simulink model "HVDCMTGW"  (R2025b)
settings: Solver=VariableStepAuto  StartTime=0.0  StopTime=Tsim  FixedStep=5e-5  RelTol=1e-3
PreLoadFcn:
  | SimulationTime = 3.5;
  | HVDCParameters;
  | Tsim = 3.5;
undefined symbols (not defined in the file): base, Base, Connection1, Connection2, Connection3, DiscIntNeverNeededParam, ee_sli_rtmsupport, frt, gcbh, grid, HVDC, lvrt, onshoreGfm, pll, pmsm, PVController, time, Ts, windController, windTransformer, windTurbine
libraries: fl_lib x51, ee_lib x46, nesl_utility x41, simulink x18, eeGeneralControl x12, eeTransforms x6
(part 1 of 4)
settings Model: SimulationMode=accelerator  Creator=Rajarshi  LastModifiedBy=rajarshd
settings SolverCC: AutoInsertRateTranBlk=on
settings DataIOCC: SaveOutput=off  DSMLogging=off  ReturnWorkspaceOutputsName=Data

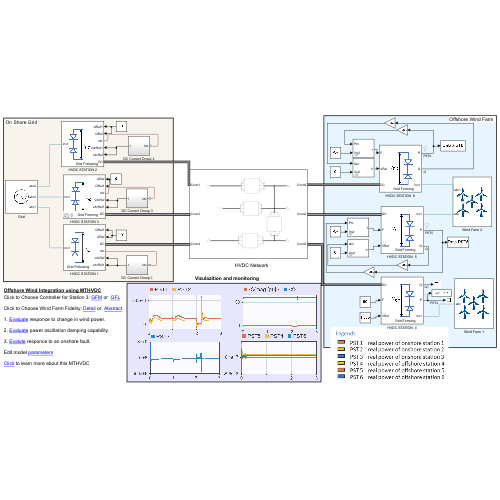
[thumbnail: Simulink's stored preview of the top-level diagram]
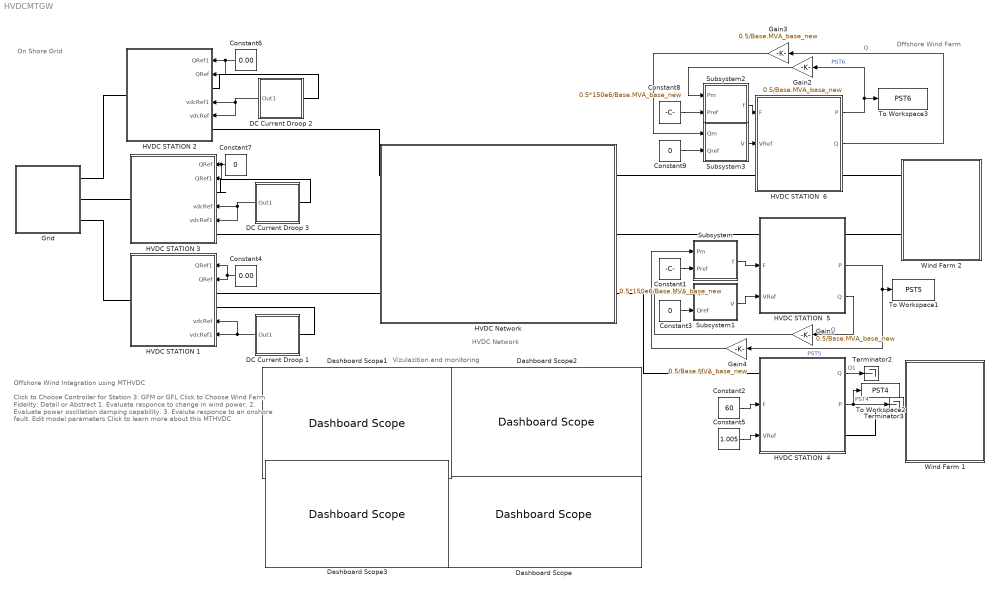
== system HVDCMTGW ==
  note: HVDC Network
  note: Click to Choose Controller for Station 3: GFM or GFL
      |
      | Click to Choose Wind Farm Fidelity: Detail or Abstract
      |
      | 1. Evaluate responce to change in wind power.
      |
      | 2. Evaluate power oscillation damping capability.
      |
      | 3. Evalute responce to an onshore fault.
      |
      | Edit model parameters
      |
      | Click to learn more about this MTHVDC
  note: Offshore Wind Integration using MTHVDC
  note: Offshore Wind Farm
  note: On Shore Grid
  note: Vizulazition and monitoring
  Constant1 : Constant  Value=0.5*150e6/Base.MVA_base_new
  Constant2 : Constant  Value=60
  Constant3 : Constant  Value=0
  Constant4 : Constant  Value=0.00
  Constant5 : Constant  Value=1.005
  Constant6 : Constant  Value=0.00
  Constant7 : Constant  Value=0
  Constant8 : Constant  Value=0.5*150e6/Base.MVA_base_new
  Constant9 : Constant  Value=0
  DC Current Droop 1 : Subsystem
  DC Current Droop 2 : Subsystem
  DC Current Droop 3 : Subsystem
  Dashboard Scope{,1..3} (4 alike) : DashboardScope  FontColor=[0.0, 0.0, 0.0]
  Gain{1..4} (4 alike) : Gain  Gain=0.5/Base.MVA_base_new
  Grid : Subsystem
  HVDC Network : Subsystem
  HVDC STATION  4 : Subsystem
      settings: PortSchema="{\"entries\":[{\"content\":{\"sides\":[{\"content\":{\"connectorIds\":[\"LConn1\",\"In1\",\"In2\"]},\"type\":\"ConnectorPlacement.EquallySpacedRectSide\",\"uuid\":\"6966c343-33fe-49bf-a40f-735765742aa3\"},{\"content\":{\"connectorIds\":[\"Out1\",\"Out2\",\"RConn1\"],\"side\":\"RIGHT\"},\"type\":\"ConnectorPlacement.EquallySpacedRectSide\",\"uuid\":\"561f8608-e59c-4a25-b590-fef3ac618496\"},{\"content\":{\"side\":\"TOP\"},\"type\":\"ConnectorPlacement.EquallySpacedRectSide\",\"uuid\":\"8731cc78-5557-4266-b8ae-4cd94a3cb230\"}]},\"type\":\"ConnectorPlacement.EquallySpacedConnector\",\"uuid\":\"a72f596e-11e5-4094-bfc9-f49a91172650\"}],\"packageUris\":[\"http://schema.mathworks.com/mf0/Connector/R2020b\"],\"version\":\"1.0\"}"
      mask Display:
      | text(40,10, 'Grid Forming');
      | image('HVDCstation.png', [0,0,0,0,80,80]);
  HVDC STATION  5 : Subsystem
      settings: PortSchema="{\"entries\":[{\"content\":{\"sides\":[{\"content\":{\"connectorIds\":[\"LConn1\",\"In1\",\"In2\"]},\"type\":\"ConnectorPlacement.EquallySpacedRectSide\",\"uuid\":\"42fca73d-9b1c-4b14-af1d-17a95f3928f9\"},{\"content\":{\"connectorIds\":[\"RConn1\",\"Out1\",\"Out2\"],\"side\":\"RIGHT\"},\"type\":\"ConnectorPlacement.EquallySpacedRectSide\",\"uuid\":\"9128ed72-a507-450a-8a5b-bb565d329306\"},{\"content\":{\"side\":\"TOP\"},\"type\":\"ConnectorPlacement.EquallySpacedRectSide\",\"uuid\":\"7e656d19-2b54-419b-9669-320b071747a0\"}]},\"type\":\"ConnectorPlacement.EquallySpacedConnector\",\"uuid\":\"734da2a5-0bfe-48f8-afaf-e709645445a8\"}],\"packageUris\":[\"http://schema.mathworks.com/mf0/Connector/R2020b\"],\"version\":\"1.0\"}"
      mask Display:
      | text(40,10, 'Grid Forming');
      | image('HVDCstation.png', [0,0,0,0,80,80]);
  HVDC STATION  6 : Subsystem
      mask Display:
      | text(40,10, 'Grid Forming');
      | image('HVDCstation.png', [0,0,0,0,80,80]);
  HVDC STATION 1 : Subsystem
      settings: PortSchema="{\"entries\":[{\"content\":{\"sides\":[{\"content\":{\"connectorIds\":[\"In1\",\"In2\",\"LConn1\",\"LConn2\",\"In3\",\"In4\"]},\"type\":\"ConnectorPlacement.EquallySpacedRectSide\",\"uuid\":\"825870e3-6597-48fb-b44e-9cac78187e1c\"},{\"content\":{\"connectorIds\":[\"RConn1\"],\"side\":\"RIGHT\"},\"type\":\"ConnectorPlacement.EquallySpacedRectSide\",\"uuid\":\"0ccf2e17-8e04-4158-8531-c061fa3c835c\"},{\"content\":{\"side\":\"TOP\"},\"type\":\"ConnectorPlacement.EquallySpacedRectSide\",\"uuid\":\"f5f3d6c6-bb99-4c25-841e-4b6e2b2ba3c2\"}]},\"type\":\"ConnectorPlacement.EquallySpacedConnector\",\"uuid\":\"7882ba9b-b66e-421c-89fd-6c0e858bc84c\"}],\"packageUris\":[\"http://schema.mathworks.com/mf0/Connector/R2020b\"],\"version\":\"1.0\"}"
      mask Display:
      | text(10,10, 'Grid Following');
      | image('HVDCstation1.png', [0,2,12,2,80,80]);
  HVDC STATION 2 : Subsystem
      settings: PortSchema="{\"entries\":[{\"content\":{\"sides\":[{\"content\":{\"connectorIds\":[\"In1\",\"In2\",\"LConn1\",\"In3\",\"In4\",\"LConn2\"]},\"type\":\"ConnectorPlacement.EquallySpacedRectSide\",\"uuid\":\"ae8d0010-9935-44cd-9427-2860d952f744\"},{\"content\":{\"connectorIds\":[\"RConn1\"],\"side\":\"RIGHT\"},\"type\":\"ConnectorPlacement.EquallySpacedRectSide\",\"uuid\":\"5b1bea21-e058-4721-9c71-335e968af1dc\"},{\"content\":{\"side\":\"TOP\"},\"type\":\"ConnectorPlacement.EquallySpacedRectSide\",\"uuid\":\"e2b4b649-cbe9-452b-9e7c-c313a834e66c\"}]},\"type\":\"ConnectorPlacement.EquallySpacedConnector\",\"uuid\":\"ef58559f-fad3-48cf-8f32-7426dfcc4f07\"}],\"packageUris\":[\"http://schema.mathworks.com/mf0/Connector/R2020b\"],\"version\":\"1.0\"}"
      mask Display:
      | text(40,10, 'Grid Following');
      | image('HVDCstation1.png', [0,2,12,2,80,80]);
  HVDC STATION 3 : Subsystem  Variant=on  mask{Choice=GFM}
      mask prompts: Choice "Controller"
      settings: PortSchema="{\"entries\":[{\"content\":{\"sides\":[{\"content\":{\"connectorIds\":[\"In1\",\"In2\",\"LConn1\",\"In3\",\"In4\",\"LConn2\"]},\"type\":\"ConnectorPlacement.EquallySpacedRectSide\",\"uuid\":\"ae8d0010-9935-44cd-9427-2860d952f744\"},{\"content\":{\"connectorIds\":[\"RConn1\"],\"side\":\"RIGHT\"},\"type\":\"ConnectorPlacement.EquallySpacedRectSide\",\"uuid\":\"5b1bea21-e058-4721-9c71-335e968af1dc\"},{\"content\":{\"side\":\"TOP\"},\"type\":\"ConnectorPlacement.EquallySpacedRectSide\",\"uuid\":\"e2b4b649-cbe9-452b-9e7c-c313a834e66c\"}]},\"type\":\"ConnectorPlacement.EquallySpacedConnector\",\"uuid\":\"ef58559f-fad3-48cf-8f32-7426dfcc4f07\"}],\"packageUris\":[\"http://schema.mathworks.com/mf0/Connector/R2020b\"],\"version\":\"1.0\"}"
  Subsystem : Subsystem  mask{kp=0.02, t=5e-3, f=60}
      mask prompts: kp "Frequency Droop (PU)"; t "Filter Time Constant (sec)"; f "Reference Frequency (Hz)"
  Subsystem1 : Subsystem  mask{kq=0.02, t=5e-3, V=1.005}
      mask prompts: kq "Voltage Droop (PU)"; t "Filter Time Constant (sec)"; V "Voltage Reference (PU)"
  Subsystem2 : Subsystem  mask{kp=0.01, t=5e-3, f=60}
      mask prompts: kp "Frequency Droop (PU)"; t "Filter Time Constant (sec)"; f "Reference Frequency (Hz)"
  Subsystem3 : Subsystem  mask{kq=0.01, t=5e-3, V=1.005}
      mask prompts: kq "Voltage Droop (PU)"; t "Filter Time Constant (sec)"; V "Voltage Reference (PU)"
  Terminator2 : Terminator
  Terminator3 : Terminator
  To Workspace1 : ToWorkspace  VariableName=PST5  SaveFormat=Timeseries  SampleTime=-1
  To Workspace2 : ToWorkspace  VariableName=PST4  SaveFormat=Timeseries  SampleTime=-1
  To Workspace3 : ToWorkspace  VariableName=PST6  SaveFormat=Timeseries  SampleTime=-1
  Wind Farm 1 : Subsystem
      mask Display: image('Windfirm3.png', [0,0,0,0,80,80]);
  Wind Farm 2 : Subsystem
      mask Display: image('Windfirm3.png', [0,0,0,0,80,80]);
  wires:
  Constant5/1 -> HVDC STATION  4/2(VRef)
  HVDC STATION  4/1(Q) -> Terminator2/1  "Q1"
  Constant2/1 -> HVDC STATION  4/1(F)
  HVDC STATION  4/2(P) -> Terminator3/1, To Workspace2/1  "PST4"
  Constant7/1 -> HVDC STATION 3/1(QRef), HVDC STATION 3/2(QRef1)
  DC Current Droop 1/1(Out1) -> HVDC STATION 1/3(vdcRef), HVDC STATION 1/4(vdcRef1)
  Constant4/1 -> HVDC STATION 1/1(QRef1), HVDC STATION 1/2(QRef)
  Constant6/1 -> HVDC STATION 2/2(QRef), HVDC STATION 2/1(QRef1)
  DC Current Droop 2/1(Out1) -> HVDC STATION 2/4(vdcRef), HVDC STATION 2/3(vdcRef1)
  Constant1/1 -> Subsystem/2(Pref)
  Constant3/1 -> Subsystem1/2(Qref)
  Constant8/1 -> Subsystem2/2(Pref)
  HVDC STATION  6/1(P) -> To Workspace3/1, Gain2/1  "PST6"
  Subsystem3/1(V) -> HVDC STATION  6/2(VRef)
  Subsystem2/1(f) -> HVDC STATION  6/1(F)
  HVDC STATION  6/2(Q) -> Gain3/1  "Q"
  Constant9/1 -> Subsystem3/2(Qref)
  Gain3/1 -> Subsystem3/1(Qm)
  Gain2/1 -> Subsystem2/1(Pm)
  Subsystem/1(f) -> HVDC STATION  5/1(F)
  Subsystem1/1(V) -> HVDC STATION  5/2(VRef)
  HVDC STATION  5/2(Q) -> Gain1/1  "Q"
  HVDC STATION  5/1(P) -> To Workspace1/1, Gain4/1  "PST5"
  Gain1/1 -> Subsystem1/1(Qm)
  Gain4/1 -> Subsystem/1(Pm)
  DC Current Droop 3/1(Out1) -> HVDC STATION 3/3(vdcRef), HVDC STATION 3/4(vdcRef1)
  connections:
  Wind Farm 2/RConn2 -- HVDC STATION  5/RConn1
  HVDC STATION 3/LConn2 -- HVDC Network/RConn2
  HVDC Network/LConn3 -- HVDC STATION  4/LConn1
  HVDC STATION 1/LConn1 -- HVDC Network/RConn3
  Grid/RConn3 -- HVDC STATION 1/RConn1
  DC Current Droop 1/LConn1 -- HVDC STATION 1/LConn2
  DC Current Droop 2/LConn1 -- HVDC STATION 2/LConn1
  HVDC STATION 2/LConn2 -- HVDC Network/RConn1
  Grid/RConn1 -- HVDC STATION 2/RConn1
  HVDC STATION  6/RConn1 -- Wind Farm 2/RConn1
  HVDC STATION  6/LConn1 -- HVDC Network/LConn1
  Wind Farm 1/RConn1 -- HVDC STATION  4/RConn1
  HVDC STATION 3/LConn1 -- DC Current Droop 3/LConn1
  HVDC STATION  5/LConn1 -- HVDC Network/LConn2
  HVDC STATION 3/RConn1 -- Grid/RConn2

== system HVDCMTGW/DC Current Droop 1 ==
  Constant : Constant  Value=HVDC.Vdc
  Gain : Gain  Gain=0.04
  Gain1 : Gain  Gain=2
  PS-Simulink Converter : nesl_utility/PS-Simulink Converter  PhysicalDomain=network_engine_domain  SubClassName=ps_output  LeftPortType=input  RightPortType=output  PseudoPeriodic=off  Frequencies=[]  VectorFormat=inherit  Unit=inherit  AffineConversion=off
  Sum : Sum  Inputs=|++
  Terminator1 : Terminator
  Unit Delay9 : UnitDelay  SampleTime=-1  HasFrameUpgradeWarning=on
  Idc : PMIOPort  Side=Left
  Out1 : Outport
  wires:
  Gain/1 -> Sum/1
  Unit Delay9/1 -> Gain/1
  Constant/1 -> Sum/2
  PS-Simulink Converter/1 -> Unit Delay9/1
  Sum/1 -> Gain1/1, Out1/1
  Gain1/1 -> Terminator1/1  "VdcRef"
  connections:
  Idc/RConn1 -- PS-Simulink Converter/LConn1

== system HVDCMTGW/DC Current Droop 2 ==
  Constant : Constant  Value=HVDC.Vdc
  Gain : Gain  Gain=0.01
  Gain1 : Gain  Gain=2
  PS-Simulink Converter : nesl_utility/PS-Simulink Converter  PhysicalDomain=network_engine_domain  SubClassName=ps_output  LeftPortType=input  RightPortType=output  PseudoPeriodic=off  Frequencies=[]  VectorFormat=inherit  Unit=inherit  AffineConversion=off
  Sum : Sum  Inputs=|++
  Terminator1 : Terminator
  Unit Delay9 : UnitDelay  SampleTime=-1  HasFrameUpgradeWarning=on
  Idc : PMIOPort  Side=Left
  Out1 : Outport
  wires:
  Gain/1 -> Sum/1
  Unit Delay9/1 -> Gain/1
  Constant/1 -> Sum/2
  PS-Simulink Converter/1 -> Unit Delay9/1
  Sum/1 -> Gain1/1, Out1/1
  Gain1/1 -> Terminator1/1  "VdcRef"
  connections:
  Idc/RConn1 -- PS-Simulink Converter/LConn1

== system HVDCMTGW/DC Current Droop 3 ==
  Constant : Constant  Value=HVDC.Vdc
  Gain : Gain  Gain=0.01
  Gain1 : Gain  Gain=2
  PS-Simulink Converter : nesl_utility/PS-Simulink Converter  PhysicalDomain=network_engine_domain  SubClassName=ps_output  LeftPortType=input  RightPortType=output  PseudoPeriodic=off  Frequencies=[]  VectorFormat=inherit  Unit=inherit  AffineConversion=off
  Sum : Sum  Inputs=|++
  Terminator1 : Terminator
  Unit Delay9 : UnitDelay  SampleTime=-1  HasFrameUpgradeWarning=on
  Idc : PMIOPort  Side=Left
  Out1 : Outport
  wires:
  Gain/1 -> Sum/1
  Unit Delay9/1 -> Gain/1
  Constant/1 -> Sum/2
  PS-Simulink Converter/1 -> Unit Delay9/1
  Sum/1 -> Gain1/1, Out1/1
  Gain1/1 -> Terminator1/1  "VdcRef"
  connections:
  Idc/RConn1 -- PS-Simulink Converter/LConn1

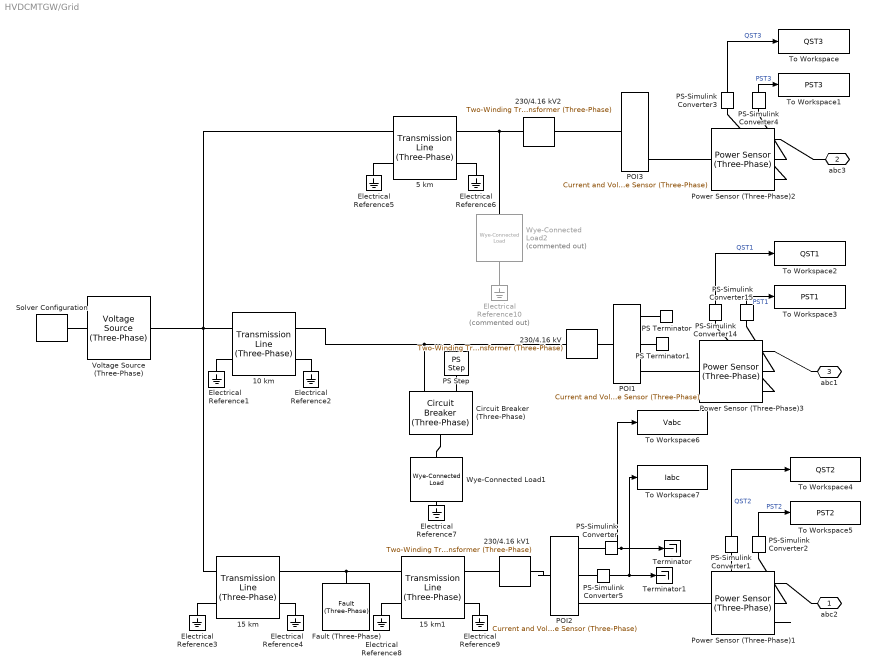
== system HVDCMTGW/Grid ==
  10 km : ee_lib/Passive/Lines/Transmission Line (Three-Phase)  length=10 km  freq=60 Hz  R=0.02 Ohm/km  L=0.5 mH/km  M=0.1 mH/km  Cl=0.3 uF/km  Cg=0.1 uF/km  Rm=0 Ohm/km  ModelTwoSections=ee.enum.enable.no  N=1  InterfacePosition=0.5 km  N1sec=1  N2sec=1  Access_ground=ee.enum.enable.no  R_parasitic=1e-6 Ohm  G_parasitic=1e-6 1/Ohm
      settings: InternalSimscapePortConfiguration="{\"Bottom\":[],\"Left\":[{\"id\":\"N1\",\"label\":\"~1\",\"type\":\"foundation.electrical.three_phase\"},{\"id\":\"g1\",\"label\":\"g1\",\"type\":\"foundation.electrical.electrical\"}],\"Right\":[{\"id\":\"N2\",\"label\":\"~2\",\"type\":\"foundation.electrical.three_phase\"},{\"id\":\"g2\",\"label\":\"g2\",\"type\":\"foundation.electrical.electrical\"}],\"Top\":[]}"
  15 km : ee_lib/Passive/Lines/Transmission Line (Three-Phase)  length=15 km  freq=60 Hz  R=0.02 Ohm/km  L=0.5 mH/km  M=0.1 mH/km  Cl=0.3 uF/km  Cg=0.1 uF/km  Rm=0 Ohm/km  ModelTwoSections=ee.enum.enable.no  N=1  InterfacePosition=0.5 km  N1sec=1  N2sec=1  Access_ground=ee.enum.enable.no  R_parasitic=1e-6 Ohm  G_parasitic=1e-6 1/Ohm
      settings: InternalSimscapePortConfiguration="{\"Bottom\":[],\"Left\":[{\"id\":\"N1\",\"label\":\"~1\",\"type\":\"foundation.electrical.three_phase\"},{\"id\":\"g1\",\"label\":\"g1\",\"type\":\"foundation.electrical.electrical\"}],\"Right\":[{\"id\":\"N2\",\"label\":\"~2\",\"type\":\"foundation.electrical.three_phase\"},{\"id\":\"g2\",\"label\":\"g2\",\"type\":\"foundation.electrical.electrical\"}],\"Top\":[]}"
  15 km1 : ee_lib/Passive/Lines/Transmission Line (Three-Phase)  length=15 km  freq=60 Hz  R=0.02 Ohm/km  L=0.5 mH/km  M=0.1 mH/km  Cl=0.3 uF/km  Cg=0.1 uF/km  Rm=0 Ohm/km  ModelTwoSections=ee.enum.enable.no  N=1  InterfacePosition=0.5 km  N1sec=1  N2sec=1  Access_ground=ee.enum.enable.no  R_parasitic=1e-6 Ohm  G_parasitic=1e-6 1/Ohm
      settings: InternalSimscapePortConfiguration="{\"Bottom\":[],\"Left\":[{\"id\":\"N1\",\"label\":\"~1\",\"type\":\"foundation.electrical.three_phase\"},{\"id\":\"g1\",\"label\":\"g1\",\"type\":\"foundation.electrical.electrical\"}],\"Right\":[{\"id\":\"N2\",\"label\":\"~2\",\"type\":\"foundation.electrical.three_phase\"},{\"id\":\"g2\",\"label\":\"g2\",\"type\":\"foundation.electrical.electrical\"}],\"Top\":[]}"
  230/4.16 kV : ee_lib/Passive/Transformers/Two-Winding Transformer (Three-Phase)  SRated=windTransformer.va A*V  FRated=grid.frequency Hz  Winding1Connection=ee.enum.windingconnection.Yg  VRated1=windTransformer.hv*1.25 V  Winding2Connection=ee.enum.windingconnection.Yg  VRated2=base.kV V  CoreType=ee.enum.coretype.threelimb  pu_Rw1=windTransformer.windingResistance/20  pu_Rw2=windTransformer.windingResistance/20  leakage_reactance_option=ee.enum.transformer_leakage.include  pu_Xl1=windTransformer.windingLekageReactance/20  pu_Xl2=windTransformer.windingLekageReactance/20  magnetizing_resistance_option=ee.enum.transformer_magnetizingResistance.exclude  pu_Rm=500  magnetizing_reactance_option=ee.enum.transformer_magnetizingReactance.exclude  saturation_option=ee.enum.transformer_saturation.exclude  pu_Xm=500  current_data=[0, .002, 1, 2]  magnetic_flux_data=[0, 1.2, 1.5, 1.51]  pu_X0=windTransformer.zeroSequenceReactance  i1_specify=off  i1_priority=None  i1=[0, 0, 0] A  i1_nominal_specify=off  i1_nominal_value=1  i1_nominal_unit=A  i2_specify=off  i2_priority=None  i2=[0, 0, 0] A  i2_nominal_specify=off  i2_nominal_value=1  i2_nominal_unit=A  phi_specify=off  phi_priority=None  phi=[0, 0, 0]  phi_nominal_specify=off  phi_nominal_value=1  phi_nominal_unit=1  power_dissipated_specify=off  power_dissipated_priority=None  power_dissipated=0 W  power_dissipated_nominal_specify=off  power_dissipated_nominal_value=1  power_dissipated_nominal_unit=W
      settings: InternalSimscapePortConfiguration="{\"Bottom\":[],\"Left\":[{\"id\":\"N1\",\"label\":\"~1\",\"type\":\"foundation.electrical.three_phase\"}],\"Right\":[{\"id\":\"N2\",\"label\":\"~2\",\"type\":\"foundation.electrical.three_phase\"}],\"Top\":[]}"
  230/4.16 kV1 : ee_lib/Passive/Transformers/Two-Winding Transformer (Three-Phase)  SRated=windTransformer.va A*V  FRated=grid.frequency Hz  Winding1Connection=ee.enum.windingconnection.Yg  VRated1=windTransformer.hv*1.25 V  Winding2Connection=ee.enum.windingconnection.Yg  VRated2=base.kV V  CoreType=ee.enum.coretype.threelimb  pu_Rw1=windTransformer.windingResistance/20  pu_Rw2=windTransformer.windingResistance/20  leakage_reactance_option=ee.enum.transformer_leakage.include  pu_Xl1=windTransformer.windingLekageReactance/20  pu_Xl2=windTransformer.windingLekageReactance/20  magnetizing_resistance_option=ee.enum.transformer_magnetizingResistance.exclude  pu_Rm=500  magnetizing_reactance_option=ee.enum.transformer_magnetizingReactance.exclude  saturation_option=ee.enum.transformer_saturation.exclude  pu_Xm=500  current_data=[0, .002, 1, 2]  magnetic_flux_data=[0, 1.2, 1.5, 1.51]  pu_X0=windTransformer.zeroSequenceReactance  i1_specify=off  i1_priority=None  i1=[0, 0, 0] A  i1_nominal_specify=off  i1_nominal_value=1  i1_nominal_unit=A  i2_specify=off  i2_priority=None  i2=[0, 0, 0] A  i2_nominal_specify=off  i2_nominal_value=1  i2_nominal_unit=A  phi_specify=off  phi_priority=None  phi=[0, 0, 0]  phi_nominal_specify=off  phi_nominal_value=1  phi_nominal_unit=1  power_dissipated_specify=off  power_dissipated_priority=None  power_dissipated=0 W  power_dissipated_nominal_specify=off  power_dissipated_nominal_value=1  power_dissipated_nominal_unit=W
      settings: InternalSimscapePortConfiguration="{\"Bottom\":[],\"Left\":[{\"id\":\"N1\",\"label\":\"~1\",\"type\":\"foundation.electrical.three_phase\"}],\"Right\":[{\"id\":\"N2\",\"label\":\"~2\",\"type\":\"foundation.electrical.three_phase\"}],\"Top\":[]}"
  230/4.16 kV2 : ee_lib/Passive/Transformers/Two-Winding Transformer (Three-Phase)  SRated=windTransformer.va A*V  FRated=grid.frequency Hz  Winding1Connection=ee.enum.windingconnection.Yg  VRated1=windTransformer.hv*1.25 V  Winding2Connection=ee.enum.windingconnection.Yg  VRated2=base.kV V  CoreType=ee.enum.coretype.threelimb  pu_Rw1=windTransformer.windingResistance/20  pu_Rw2=windTransformer.windingResistance/20  leakage_reactance_option=ee.enum.transformer_leakage.include  pu_Xl1=windTransformer.windingLekageReactance/20  pu_Xl2=windTransformer.windingLekageReactance/20  magnetizing_resistance_option=ee.enum.transformer_magnetizingResistance.exclude  pu_Rm=500  magnetizing_reactance_option=ee.enum.transformer_magnetizingReactance.exclude  saturation_option=ee.enum.transformer_saturation.exclude  pu_Xm=500  current_data=[0, .002, 1, 2]  magnetic_flux_data=[0, 1.2, 1.5, 1.51]  pu_X0=windTransformer.zeroSequenceReactance  i1_specify=off  i1_priority=None  i1=[0, 0, 0] A  i1_nominal_specify=off  i1_nominal_value=1  i1_nominal_unit=A  i2_specify=off  i2_priority=None  i2=[0, 0, 0] A  i2_nominal_specify=off  i2_nominal_value=1  i2_nominal_unit=A  phi_specify=off  phi_priority=None  phi=[0, 0, 0]  phi_nominal_specify=off  phi_nominal_value=1  phi_nominal_unit=1  power_dissipated_specify=off  power_dissipated_priority=None  power_dissipated=0 W  power_dissipated_nominal_specify=off  power_dissipated_nominal_value=1  power_dissipated_nominal_unit=W
      settings: InternalSimscapePortConfiguration="{\"Bottom\":[],\"Left\":[{\"id\":\"N1\",\"label\":\"~1\",\"type\":\"foundation.electrical.three_phase\"}],\"Right\":[{\"id\":\"N2\",\"label\":\"~2\",\"type\":\"foundation.electrical.three_phase\"}],\"Top\":[]}"
  5 km : ee_lib/Passive/Lines/Transmission Line (Three-Phase)  length=5 km  freq=60 Hz  R=0.02 Ohm/km  L=0.5 mH/km  M=0.1 mH/km  Cl=0.3 uF/km  Cg=0.1 uF/km  Rm=0 Ohm/km  ModelTwoSections=ee.enum.enable.no  N=1  InterfacePosition=0.5 km  N1sec=1  N2sec=1  Access_ground=ee.enum.enable.no  R_parasitic=1e-6 Ohm  G_parasitic=1e-6 1/Ohm
      settings: InternalSimscapePortConfiguration="{\"Bottom\":[],\"Left\":[{\"id\":\"N1\",\"label\":\"~1\",\"type\":\"foundation.electrical.three_phase\"},{\"id\":\"g1\",\"label\":\"g1\",\"type\":\"foundation.electrical.electrical\"}],\"Right\":[{\"id\":\"N2\",\"label\":\"~2\",\"type\":\"foundation.electrical.three_phase\"},{\"id\":\"g2\",\"label\":\"g2\",\"type\":\"foundation.electrical.electrical\"}],\"Top\":[]}"
  Circuit Breaker (Three-Phase) : ee_lib/Switches & Breakers/Circuit Breaker (Three-Phase)  R_closed=1e-7 Ohm  G_open=1e-6 1/Ohm  threshold=0.5 V  breaker_behavior=ee.enum.switches.breakerBehavior.zeroCrossingDisable
      settings: InternalSimscapePortConfiguration="{\"Bottom\":[],\"Left\":[{\"id\":\"vT\",\"label\":\"vT\",\"type\":\"input\"},{\"id\":\"N1\",\"label\":\"~1\",\"type\":\"foundation.electrical.three_phase\"}],\"Right\":[{\"id\":\"N2\",\"label\":\"~2\",\"type\":\"foundation.electrical.three_phase\"}],\"Top\":[]}"
  Electrical Reference{1..9} (9 alike) : fl_lib/Electrical/Electrical Elements/Electrical Reference
  Electrical Reference10 : fl_lib/Electrical/Electrical Elements/Electrical Reference  Commented=on
  Fault (Three-Phase) : ee_lib/Utilities/Fault (Three-Phase)  fault_type_option=11  R_pn_fault=1e-6 Ohm  R_ng_fault=1e-6 Ohm  exposemeasurement=ee.enum.exposemeasurement.hidden  enable_external_fault=ee.enum.external_fault.hidden  fault_threshold=0.5  fault_condition=1  fault_resettable=0  enable_temporal_fault=1  fault_start_time=time.fault s  fault_duration=0.2 s  G_parasitic=1e-6 1/Ohm
      settings: InternalSimscapePortConfiguration="{\"Bottom\":[],\"Left\":[{\"id\":\"N\",\"label\":\"~\",\"type\":\"foundation.electrical.three_phase\"}],\"Right\":[],\"Top\":[]}"
  POI1 : ee_lib/Sensors & Transducers/Current and Voltage Sensor (Three-Phase)  vMeasurementType=ee.enum.vmeasurement.lg  outputUnit=ee.enum.unit.pu  SRated=Base.MVA_base_new A*V  VRated=base.kV V  I_specify=off  I_priority=None  I=[0, 0, 0] A  I_nominal_specify=off  I_nominal_value=1  I_nominal_unit=A  V_specify=off  V_priority=None  V=[0, 0, 0] V  V_nominal_specify=off  V_nominal_value=1  V_nominal_unit=V
      settings: InternalSimscapePortConfiguration="{\"Bottom\":[],\"Left\":[{\"id\":\"N1\",\"label\":\"~1\",\"type\":\"foundation.electrical.three_phase\"}],\"Right\":[{\"id\":\"V_output\",\"label\":\"V\",\"type\":\"output\"},{\"id\":\"I_output\",\"label\":\"I\",\"type\":\"output\"},{\"id\":\"N2\",\"label\":\"~2\",\"type\":\"foundation.electrical.three_phase\"}],\"Top\":[]}"
  POI2 : ee_lib/Sensors & Transducers/Current and Voltage Sensor (Three-Phase)  vMeasurementType=ee.enum.vmeasurement.lg  outputUnit=ee.enum.unit.pu  SRated=Base.MVA_base_new A*V  VRated=base.kV V  I_specify=off  I_priority=None  I=[0, 0, 0] A  I_nominal_specify=off  I_nominal_value=1  I_nominal_unit=A  V_specify=off  V_priority=None  V=[0, 0, 0] V  V_nominal_specify=off  V_nominal_value=1  V_nominal_unit=V
      settings: InternalSimscapePortConfiguration="{\"Bottom\":[],\"Left\":[{\"id\":\"N1\",\"label\":\"~1\",\"type\":\"foundation.electrical.three_phase\"}],\"Right\":[{\"id\":\"V_output\",\"label\":\"V\",\"type\":\"output\"},{\"id\":\"I_output\",\"label\":\"I\",\"type\":\"output\"},{\"id\":\"N2\",\"label\":\"~2\",\"type\":\"foundation.electrical.three_phase\"}],\"Top\":[]}"
  POI3 : ee_lib/Sensors & Transducers/Current and Voltage Sensor (Three-Phase)  vMeasurementType=ee.enum.vmeasurement.lg  outputUnit=ee.enum.unit.pu  SRated=Base.MVA_base_new A*V  VRated=base.kV V  I_specify=off  I_priority=None  I=[0, 0, 0] A  I_nominal_specify=off  I_nominal_value=1  I_nominal_unit=A  V_specify=off  V_priority=None  V=[0, 0, 0] V  V_nominal_specify=off  V_nominal_value=1  V_nominal_unit=V
      settings: InternalSimscapePortConfiguration="{\"Bottom\":[],\"Left\":[{\"id\":\"N1\",\"label\":\"~1\",\"type\":\"foundation.electrical.three_phase\"}],\"Right\":[{\"id\":\"V_output\",\"label\":\"V\",\"type\":\"output\"},{\"id\":\"I_output\",\"label\":\"I\",\"type\":\"output\"},{\"id\":\"N2\",\"label\":\"~2\",\"type\":\"foundation.electrical.three_phase\"}],\"Top\":[]}"
  PS Step : fl_lib/Physical Signals/Sources/PS Step  step_time=time.load s  initial_value=0  final_value=1
  PS Terminator : fl_lib/Physical Signals/Sinks/PS Terminator
  PS Terminator1 : fl_lib/Physical Signals/Sinks/PS Terminator
  PS-Simulink Converter{,1..5,14..15} (8 alike) : nesl_utility/PS-Simulink Converter  PhysicalDomain=network_engine_domain  SubClassName=ps_output  LeftPortType=input  RightPortType=output  PseudoPeriodic=off  Frequencies=[]  VectorFormat=inherit  Unit=inherit  AffineConversion=off
  Power Sensor (Three-Phase)1 : ee_lib/Sensors & Transducers/Power Sensor (Three-Phase)  load_type=ee.enum.passive.type_balanced.balanced  f0=60 Hz
      settings: InternalSimscapePortConfiguration="{\"Bottom\":[],\"Left\":[{\"id\":\"N1\",\"label\":\"~1\",\"type\":\"foundation.electrical.three_phase\"}],\"Right\":[{\"id\":\"N2\",\"label\":\"~2\",\"type\":\"foundation.electrical.three_phase\"}],\"Top\":[{\"id\":\"Pm\",\"label\":\"P\",\"type\":\"output\"},{\"id\":\"Qm\",\"label\":\"Q\",\"type\":\"output\"}]}"
  Power Sensor (Three-Phase)2 : ee_lib/Sensors & Transducers/Power Sensor (Three-Phase)  load_type=ee.enum.passive.type_balanced.balanced  f0=60 Hz
      settings: InternalSimscapePortConfiguration="{\"Bottom\":[],\"Left\":[{\"id\":\"N1\",\"label\":\"~1\",\"type\":\"foundation.electrical.three_phase\"}],\"Right\":[{\"id\":\"N2\",\"label\":\"~2\",\"type\":\"foundation.electrical.three_phase\"}],\"Top\":[{\"id\":\"Pm\",\"label\":\"P\",\"type\":\"output\"},{\"id\":\"Qm\",\"label\":\"Q\",\"type\":\"output\"}]}"
  Power Sensor (Three-Phase)3 : ee_lib/Sensors & Transducers/Power Sensor (Three-Phase)  load_type=ee.enum.passive.type_balanced.balanced  f0=60 Hz
      settings: InternalSimscapePortConfiguration="{\"Bottom\":[],\"Left\":[{\"id\":\"N1\",\"label\":\"~1\",\"type\":\"foundation.electrical.three_phase\"}],\"Right\":[{\"id\":\"N2\",\"label\":\"~2\",\"type\":\"foundation.electrical.three_phase\"}],\"Top\":[{\"id\":\"Pm\",\"label\":\"P\",\"type\":\"output\"},{\"id\":\"Qm\",\"label\":\"Q\",\"type\":\"output\"}]}"
  Solver Configuration : nesl_utility/Solver Configuration  PhysicalDomain=network_engine_domain  SubClassName=solver  LeftPortType=input  RightPortType=generic  Tones=[]  Harmonics=[]  SimulateNoise=off  Profile=off  UseLocalSampling=off  EnableSwitchedLinearOptims=on  FrequencyDomain=off  UseCCode=off  RelTol=0.001  AbsTol=0.001  MinStep=1e-09  ToWorkspace=off  RevertToSquareIcSolve=off  NumHomotopyIterations=100  PhasorMode=off  PhasorModeNumHarmonics=1  ConsistencySolver=NEWTON_XTOL_AFTER_FTOL  IndexReductionMethod=None  DoDC=off  ResidualTolerance=1e-09  ConsistencyTolSource=LOCAL  ConsistencyAbsTol=1e-3  ConsistencyRelTol=1e-3  ConsistencyTolFactor=1e-3  UseLocalSolver=on  LocalSolverChoice=NE_BACKWARD_EULER_ADVANCER  ResolveIndetEquations=off  FunctionEvalNumThread=1  LocalSolverSampleTime=5e-5  DoFixedCost=on  MaxNonlinIter=1  MaxModeIter=2  ComputeImpulses=off  ImpulseIterations=2  LinearAlgebra=Sparse  LinearAlgebraNumThread=0  EquationFormulation=NE_TIME_EF  DelaysMemoryBudget=1024  AutomaticFiltering=off  FilteringTimeConstant=0.001  PartitionStorageMethod=AS_NEEDED  PartitionMemoryBudget=1024  PartitionMethod=ROBUST  MultibodyUseLocalSolver=off  MultibodyLocalSolverChoice=ODE1  MultibodyLocalSolverSampleTime=0.001
  Terminator : Terminator
  Terminator1 : Terminator
  To Workspace : ToWorkspace  VariableName=QST3  SaveFormat=Timeseries  SampleTime=-1
  To Workspace1 : ToWorkspace  VariableName=PST3  SaveFormat=Timeseries  SampleTime=-1
  To Workspace2 : ToWorkspace  VariableName=QST1  SaveFormat=Timeseries  SampleTime=-1
  To Workspace3 : ToWorkspace  VariableName=PST1  SaveFormat=Timeseries  SampleTime=-1
  To Workspace4 : ToWorkspace  VariableName=QST2  SaveFormat=Timeseries  SampleTime=-1
  To Workspace5 : ToWorkspace  VariableName=PST2  SaveFormat=Timeseries  SampleTime=-1
  To Workspace6 : ToWorkspace  VariableName=Vabc  SaveFormat=Timeseries  SampleTime=-1
  To Workspace7 : ToWorkspace  VariableName=Iabc  SaveFormat=Timeseries  SampleTime=-1
  Voltage Source (Three-Phase) : ee_lib/Sources/Voltage Source (Three-Phase)  vline_rms=Grid.voltage V  shift=0 deg  freq=Grid.frequency Hz  impedance_option=4  SShortCircuit=1e6 A*V  XR=15  R=grid.rs*1.2 Ohm  L=grid.ls*1.2 H  harmonic_option=0  harmonic_orders=[5, 7, 11, 13]  harmonic_ratios=[.1, .1, .1, .1]  G_parasitic=1e-6 1/Ohm  I_specify=off  I_priority=None  I=[0, 0, 0] A  I_nominal_specify=off  I_nominal_value=1  I_nominal_unit=A
  Wye-Connected Load1 : ee_lib/Passive/RLC Assemblies/Wye-Connected Load  port_option=ee.enum.threePhasePort.composite  parameterization=ee.enum.rlc.parameterization.ratedpower  component_structure=ee.enum.rlc.structure.R  component_structure_PQ=ee.enum.rlc.structure.R  R=1 Ohm  L=1e-3 H  C=1e-6 F  VRated=230e3 V  FRated=60 Hz  P=300 MW  Qpos=100 A*V  Qneg=-1e2 A*V  R_parasitic=0 Ohm  G_parasitic=0 1/Ohm  R_parasitic_PQ=0 Ohm  G_parasitic_PQ=1e-9 1/Ohm  Vmag0=230e3 V  Vang0=0 deg  Freq0=60 Hz  IL_specify=off  IL_priority=High  IL=[0, 0, 0] A  IL_nominal_specify=off  IL_nominal_value=1  IL_nominal_unit=A  VC_specify=off  VC_priority=High  VC=[0, 0, 0] V  VC_nominal_specify=off  VC_nominal_value=1  VC_nominal_unit=V
  Wye-Connected Load2 : ee_lib/Passive/RLC Assemblies/Wye-Connected Load  Commented=on  port_option=ee.enum.threePhasePort.composite  parameterization=ee.enum.rlc.parameterization.ratedpower  component_structure=ee.enum.rlc.structure.R  component_structure_PQ=ee.enum.rlc.structure.R  R=1 Ohm  L=1e-3 H  C=1e-6 F  VRated=230e3 V  FRated=60 Hz  P=100 MW  Qpos=100 A*V  Qneg=-1e2 A*V  R_parasitic=0 Ohm  G_parasitic=0 1/Ohm  R_parasitic_PQ=0 Ohm  G_parasitic_PQ=1e-9 1/Ohm  Vmag0=230e3 V  Vang0=0 deg  Freq0=60 Hz  IL_specify=off  IL_priority=High  IL=[0, 0, 0] A  IL_nominal_specify=off  IL_nominal_value=1  IL_nominal_unit=A  VC_specify=off  VC_priority=High  VC=[0, 0, 0] V  VC_nominal_specify=off  VC_nominal_value=1  VC_nominal_unit=V
  abc2 : PMIOPort  Side=Right
  abc3 : PMIOPort  Port=2  Side=Right
  abc1 : PMIOPort  Port=3  Side=Right
  wires:
  PS-Simulink Converter3/1 -> To Workspace/1  "QST3"
  PS-Simulink Converter4/1 -> To Workspace1/1  "PST3"
  PS-Simulink Converter15/1 -> To Workspace3/1  "PST1"
  PS-Simulink Converter14/1 -> To Workspace2/1  "QST1"
  PS-Simulink Converter2/1 -> To Workspace5/1  "PST2"
  PS-Simulink Converter1/1 -> To Workspace4/1  "QST2"
  PS-Simulink Converter/1 -> Terminator/1, To Workspace6/1
  PS-Simulink Converter5/1 -> To Workspace7/1, Terminator1/1
  connections:
  230/4.16 kV/RConn1 -- POI1/LConn1
  Power Sensor (Three-Phase)3/LConn2 -- PS-Simulink Converter15/LConn1
  Power Sensor (Three-Phase)3/LConn3 -- PS-Simulink Converter14/LConn1
  Electrical Reference1/LConn1 -- 10 km/LConn2
  Electrical Reference2/LConn1 -- 10 km/RConn2
  Voltage Source (Three-Phase)/RConn1 -- 5 km/LConn1 -- 15 km/LConn1 -- 10 km/LConn1
  10 km/RConn1 -- Circuit Breaker (Three-Phase)/LConn2 -- 230/4.16 kV/LConn1
  15 km1/LConn1 -- Fault (Three-Phase)/LConn1 -- 15 km/RConn1
  Electrical Reference3/LConn1 -- 15 km/LConn2
  Power Sensor (Three-Phase)1/LConn3 -- PS-Simulink Converter1/LConn1
  Power Sensor (Three-Phase)1/LConn2 -- PS-Simulink Converter2/LConn1
  Electrical Reference4/LConn1 -- 15 km/RConn2
  Electrical Reference6/LConn1 -- 5 km/RConn2
  5 km/RConn1 -- Wye-Connected Load2/LConn1 -- 230/4.16 kV2/LConn1
  Electrical Reference5/LConn1 -- 5 km/LConn2
  Power Sensor (Three-Phase)2/LConn3 -- PS-Simulink Converter3/LConn1
  Power Sensor (Three-Phase)2/LConn2 -- PS-Simulink Converter4/LConn1
  abc3/RConn1 -- Power Sensor (Three-Phase)2/LConn1
  Power Sensor (Three-Phase)3/LConn1 -- abc1/RConn1
  Power Sensor (Three-Phase)1/LConn1 -- abc2/RConn1
  POI2/LConn1 -- 230/4.16 kV1/RConn1
  POI2/RConn3 -- Power Sensor (Three-Phase)1/RConn1
  POI3/LConn1 -- 230/4.16 kV2/RConn1
  POI3/RConn3 -- Power Sensor (Three-Phase)2/RConn1
  POI1/RConn3 -- Power Sensor (Three-Phase)3/RConn1
  PS Terminator/LConn1 -- POI1/RConn1
  PS Terminator1/LConn1 -- POI1/RConn2
  Electrical Reference8/LConn1 -- 15 km1/LConn2
  15 km1/RConn1 -- 230/4.16 kV1/LConn1
  Electrical Reference9/LConn1 -- 15 km1/RConn2
  PS-Simulink Converter/LConn1 -- POI2/RConn1
  PS-Simulink Converter5/LConn1 -- POI2/RConn2
  Solver Configuration/RConn1 -- Voltage Source (Three-Phase)/LConn1
  Electrical Reference10/LConn1 -- Wye-Connected Load2/RConn1
  Circuit Breaker (Three-Phase)/RConn1 -- Wye-Connected Load1/LConn1
  Electrical Reference7/LConn1 -- Wye-Connected Load1/RConn1
  PS Step/RConn1 -- Circuit Breaker (Three-Phase)/LConn1

== system HVDCMTGW/HVDC Network ==
  DC Line 10 km : Subsystem  mask{rdc=0.02, Ldc=1.04e-3, rn=0.02, l=10}
      mask prompts: rdc "Line Resistance (Ohms/km)"; Ldc "Line Inductance (H/km)"; rn "Nutrel Resistance (Ohms/km)"; l "Line Length (km)"
      mask Display: image('Network.png', [0,0,0,0,80,80]);
  DC Line 125 km : Subsystem  mask{rdc=0.02, Ldc=1.04e-3, rn=0.02, l=125}
      mask prompts: rdc "Line Resistance (Ohms/km)"; Ldc "Line Inductance (H/km)"; rn "Nutrel Resistance (Ohms/km)"; l "Line Length (km)"
      mask Display: image('Network.png', [0,0,0,0,80,80]);
  DC Line 200 km : Subsystem  mask{rdc=0.02, Ldc=1.04e-3, rn=0.02, l=200}
      mask prompts: rdc "Line Resistance (Ohms/km)"; Ldc "Line Inductance (H/km)"; rn "Nutrel Resistance (Ohms/km)"; l "Line Length (km)"
      mask Display: image('Network.png', [0,0,0,0,80,80]);
  DC Line 205 km : Subsystem  mask{rdc=0.02, Ldc=1.04e-3, rn=0.02, l=205}
      mask prompts: rdc "Line Resistance (Ohms/km)"; Ldc "Line Inductance (H/km)"; rn "Nutrel Resistance (Ohms/km)"; l "Line Length (km)"
      mask Display: image('Network.png', [0,0,0,0,80,80]);
  Simscape Bus{1..8} (8 alike) : SimscapeBus  HierarchyStrings=Connection1;Connection2;Connection3
  Conn6 : PMIOPort  Side=Left
  Conn2 : PMIOPort  Port=2  Side=Left
  Conn5 : PMIOPort  Port=3  Side=Left
  Conn1 : PMIOPort  Port=4  Side=Right
  Conn3 : PMIOPort  Port=5  Side=Right
  Conn4 : PMIOPort  Port=6  Side=Right
  connections:
  Simscape Bus3/LConn1 -- DC Line 200 km/LConn1
  Simscape Bus4/RConn1 -- Conn6/RConn1 -- Simscape Bus6/RConn1 -- Simscape Bus7/RConn1 -- Conn2/RConn1
  Simscape Bus3/LConn3 -- DC Line 200 km/LConn3
  Simscape Bus2/LConn3 -- DC Line 125 km/RConn3
  Simscape Bus3/LConn2 -- DC Line 200 km/LConn2
  Conn1/RConn1 -- Simscape Bus3/RConn1
  Simscape Bus5/LConn2 -- DC Line 205 km/LConn2
  Simscape Bus4/LConn2 -- DC Line 200 km/RConn2
  Simscape Bus4/LConn1 -- DC Line 200 km/RConn1
  Simscape Bus4/LConn3 -- DC Line 200 km/RConn3
  Simscape Bus6/LConn3 -- DC Line 205 km/RConn3
  Simscape Bus2/LConn2 -- DC Line 125 km/RConn2
  Simscape Bus2/LConn1 -- DC Line 125 km/RConn1
  Simscape Bus8/LConn3 -- DC Line 10 km/RConn3
  Simscape Bus7/LConn3 -- DC Line 10 km/LConn3
  Simscape Bus7/LConn1 -- DC Line 10 km/LConn1
  Simscape Bus5/LConn1 -- DC Line 205 km/LConn1
  Simscape Bus6/LConn1 -- DC Line 205 km/RConn1
  Simscape Bus5/LConn3 -- DC Line 205 km/LConn3
  Simscape Bus6/LConn2 -- DC Line 205 km/RConn2
  Simscape Bus8/LConn1 -- DC Line 10 km/RConn1
  Simscape Bus2/RConn1 -- Simscape Bus8/RConn1 -- Conn5/RConn1
  Simscape Bus8/LConn2 -- DC Line 10 km/RConn2
  Simscape Bus7/LConn2 -- DC Line 10 km/LConn2
  Conn4/RConn1 -- Simscape Bus1/RConn1
  Simscape Bus1/LConn1 -- DC Line 125 km/LConn1
  Simscape Bus1/LConn2 -- DC Line 125 km/LConn2
  Simscape Bus1/LConn3 -- DC Line 125 km/LConn3
  Conn3/RConn1 -- Simscape Bus5/RConn1

== system HVDCMTGW/HVDC STATION  4 ==
  F : Inport
  VRef : Inport  Port=2
  Constant : Constant  Value=1.003
  Constant1 : Constant  Value=0
  ERef1 : fl_lib/Electrical/Electrical Elements/Electrical Reference
  Gain : Gain  Gain=1/HVDC.Vdc
  Gain1 : Gain  Gain=-500
  PS-Simulink Converter : nesl_utility/PS-Simulink Converter  PhysicalDomain=network_engine_domain  SubClassName=ps_output  LeftPortType=input  RightPortType=output  PseudoPeriodic=off  Frequencies=[]  VectorFormat=inherit  Unit=inherit  AffineConversion=off
  PS-Simulink Converter1 : nesl_utility/PS-Simulink Converter  PhysicalDomain=network_engine_domain  SubClassName=ps_output  LeftPortType=input  RightPortType=output  PseudoPeriodic=off  Frequencies=[]  VectorFormat=inherit  Unit=inherit  AffineConversion=off
  Power Sensor (Three-Phase) : ee_lib/Sensors & Transducers/Power Sensor (Three-Phase)  load_type=ee.enum.passive.type_balanced.balanced  f0=60 Hz
      settings: InternalSimscapePortConfiguration="{\"Bottom\":[],\"Left\":[{\"id\":\"N1\",\"label\":\"~1\",\"type\":\"foundation.electrical.three_phase\"}],\"Right\":[{\"id\":\"N2\",\"label\":\"~2\",\"type\":\"foundation.electrical.three_phase\"}],\"Top\":[{\"id\":\"Pm\",\"label\":\"P\",\"type\":\"output\"},{\"id\":\"Qm\",\"label\":\"Q\",\"type\":\"output\"}]}"
  Simscape Bus : SimscapeBus  HierarchyStrings=Connection1;Connection2;Connection3
  Simulink-PS Converter : nesl_utility/Simulink-PS Converter  PhysicalDomain=network_engine_domain  SubClassName=ps_input  LeftPortType=input  RightPortType=output  PseudoPeriodic=off  Frequencies=[]  NoiseDistribution=none  NoiseParameters=[]  Unit=1  AffineConversion=off  FilteringAndDerivatives=provide  SimscapeFilterOrder=1  InputFilterTimeConstant=0.001  UdotUserProvided=0
  Simulink-PS Converter1 : nesl_utility/Simulink-PS Converter  PhysicalDomain=network_engine_domain  SubClassName=ps_input  LeftPortType=input  RightPortType=output  PseudoPeriodic=off  Frequencies=[]  NoiseDistribution=none  NoiseParameters=[]  Unit=1  AffineConversion=off  FilteringAndDerivatives=provide  SimscapeFilterOrder=1  InputFilterTimeConstant=0.001  UdotUserProvided=0
  Subsystem3 : Subsystem
      settings: PortSchema="{\"entries\":[{\"content\":{\"sides\":[{\"content\":{\"connectorIds\":[\"In1\",\"In2\",\"In3\"]},\"type\":\"ConnectorPlacement.EquallySpacedRectSide\",\"uuid\":\"fdf47ade-06a3-4164-a0ae-b5ab8f0b8a55\"},{\"content\":{\"connectorIds\":[\"In4\",\"Out1\",\"Out2\"],\"side\":\"RIGHT\"},\"type\":\"ConnectorPlacement.EquallySpacedRectSide\",\"uuid\":\"e0a966ff-b656-4cbf-a7ff-a400da725053\"},{\"content\":{\"side\":\"TOP\"},\"type\":\"ConnectorPlacement.EquallySpacedRectSide\",\"uuid\":\"151062ed-8c36-492f-8148-99554d7644ec\"},{\"content\":{\"side\":\"BOTTOM\"},\"type\":\"ConnectorPlacement.EquallySpacedRectSide\",\"uuid\":\"8f8a2450-c04a-404e-aef9-a0f993b87536\"}]},\"type\":\"ConnectorPlacement.EquallySpacedConnector\",\"uuid\":\"01811104-26cd-432b-92b8-9bb1e91d8204\"}],\"packageUris\":[\"http://schema.mathworks.com/mf0/Connector/R2020b\"],\"version\":\"1.0\"}"
  Subsystem4 : Subsystem  ReferencedSubsystem=HVDCSTATION  c=HVDC.C*0.1  vc=HVDC.Vdc  L=HVDC.L/5  VRated=base.kV1  SRated=Base.MVA_base_new  t=grid.sensorTime  Ts=Ts
  Sum : Sum  Inputs=|++
  Sum1 : Sum  Inputs=|+-
  Switch : Switch  Criteria=u2 > Threshold  SaturateOnIntegerOverflow=off  InputSameDT=off
  Terminator1 : Terminator
  Terminator2 : Terminator
  Terminator3 : Terminator
  Unit Delay : UnitDelay  SampleTime=-1  HasFrameUpgradeWarning=on
  Unit Delay1 : UnitDelay  SampleTime=-1  HasFrameUpgradeWarning=on
  Unit Delay3 : UnitDelay  SampleTime=-1  HasFrameUpgradeWarning=on
  DC : PMIOPort  Side=Left
  inv1 : PMIOPort  Port=2  Side=Right
  Q : Outport
  P : Outport  Port=2
  wires:
  Subsystem4/2 -> Unit Delay/1
  Subsystem4/6 -> Terminator3/1
  Subsystem4/5 -> Unit Delay3/1
  Subsystem4/4 -> Terminator2/1
  F/1 -> Subsystem3/4(F)
  Subsystem4/3 -> Terminator1/1
  Sum/1 -> Subsystem3/3(Vref)
  VRef/1 -> Sum/1
  PS-Simulink Converter1/1 -> P/1
  PS-Simulink Converter/1 -> Q/1
  Unit Delay/1 -> Subsystem3/2(Vabc)
  Unit Delay3/1 -> Subsystem3/1(Vabc1)
  Gain/1 -> Sum1/1  "VdcOff"
  Constant/1 -> Sum1/2
  Constant1/1 -> Switch/3
  Switch/1 -> Gain1/1
  Sum1/1 -> Switch/1, Switch/2
  Gain1/1 -> Unit Delay1/1
  Unit Delay1/1 -> Sum/2
  Subsystem4/1 -> Gain/1
  Subsystem3/2(VabcRef) -> Simulink-PS Converter/1
  Subsystem3/1(VabcRef1) -> Simulink-PS Converter1/1
  connections:
  Subsystem4/LConn3 -- Simscape Bus/LConn1
  Subsystem4/LConn4 -- Simscape Bus/LConn2
  DC/RConn1 -- Simscape Bus/RConn1
  PS-Simulink Converter/LConn1 -- Power Sensor (Three-Phase)/LConn3
  Power Sensor (Three-Phase)/LConn1 -- inv1/RConn1
  Power Sensor (Three-Phase)/RConn1 -- Subsystem4/RConn1
  PS-Simulink Converter1/LConn1 -- Power Sensor (Three-Phase)/LConn2
  Subsystem4/LConn6 -- ERef1/LConn1
  Subsystem4/LConn5 -- Simscape Bus/LConn3
  Simulink-PS Converter/RConn1 -- Subsystem4/LConn1
  Simulink-PS Converter1/RConn1 -- Subsystem4/LConn2

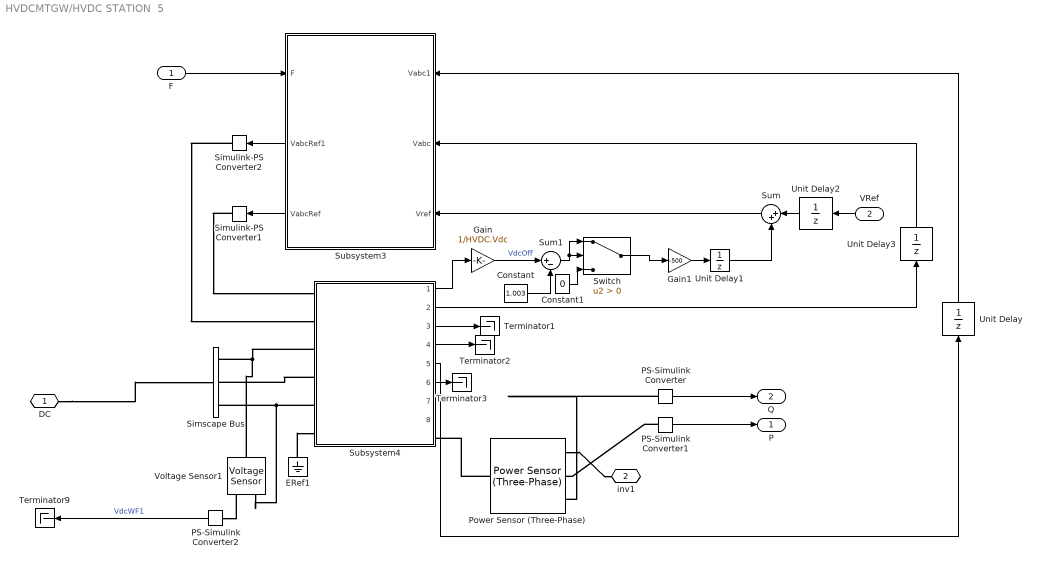
== system HVDCMTGW/HVDC STATION  5 ==
  F : Inport
  VRef : Inport  Port=2
  Constant : Constant  Value=1.003
  Constant1 : Constant  Value=0
  ERef1 : fl_lib/Electrical/Electrical Elements/Electrical Reference
  Gain : Gain  Gain=1/HVDC.Vdc
  Gain1 : Gain  Gain=-500
  PS-Simulink Converter : nesl_utility/PS-Simulink Converter  PhysicalDomain=network_engine_domain  SubClassName=ps_output  LeftPortType=input  RightPortType=output  PseudoPeriodic=off  Frequencies=[]  VectorFormat=inherit  Unit=inherit  AffineConversion=off
  PS-Simulink Converter1 : nesl_utility/PS-Simulink Converter  PhysicalDomain=network_engine_domain  SubClassName=ps_output  LeftPortType=input  RightPortType=output  PseudoPeriodic=off  Frequencies=[]  VectorFormat=inherit  Unit=inherit  AffineConversion=off
  PS-Simulink Converter2 : nesl_utility/PS-Simulink Converter  PhysicalDomain=network_engine_domain  SubClassName=ps_output  LeftPortType=input  RightPortType=output  PseudoPeriodic=off  Frequencies=[]  VectorFormat=inherit  Unit=inherit  AffineConversion=off
  Power Sensor (Three-Phase) : ee_lib/Sensors & Transducers/Power Sensor (Three-Phase)  load_type=ee.enum.passive.type_balanced.balanced  f0=60 Hz
      settings: InternalSimscapePortConfiguration="{\"Bottom\":[],\"Left\":[{\"id\":\"N1\",\"label\":\"~1\",\"type\":\"foundation.electrical.three_phase\"}],\"Right\":[{\"id\":\"N2\",\"label\":\"~2\",\"type\":\"foundation.electrical.three_phase\"}],\"Top\":[{\"id\":\"Pm\",\"label\":\"P\",\"type\":\"output\"},{\"id\":\"Qm\",\"label\":\"Q\",\"type\":\"output\"}]}"
  Simscape Bus : SimscapeBus  HierarchyStrings=Connection1;Connection2;Connection3
  Simulink-PS Converter1 : nesl_utility/Simulink-PS Converter  PhysicalDomain=network_engine_domain  SubClassName=ps_input  LeftPortType=input  RightPortType=output  PseudoPeriodic=off  Frequencies=[]  NoiseDistribution=none  NoiseParameters=[]  Unit=1  AffineConversion=off  FilteringAndDerivatives=provide  SimscapeFilterOrder=1  InputFilterTimeConstant=0.001  UdotUserProvided=0
  Simulink-PS Converter2 : nesl_utility/Simulink-PS Converter  PhysicalDomain=network_engine_domain  SubClassName=ps_input  LeftPortType=input  RightPortType=output  PseudoPeriodic=off  Frequencies=[]  NoiseDistribution=none  NoiseParameters=[]  Unit=1  AffineConversion=off  FilteringAndDerivatives=provide  SimscapeFilterOrder=1  InputFilterTimeConstant=0.001  UdotUserProvided=0
  Subsystem3 : Subsystem
      settings: PortSchema="{\"entries\":[{\"content\":{\"sides\":[{\"content\":{\"connectorIds\":[\"In1\",\"In2\",\"In3\"]},\"type\":\"ConnectorPlacement.EquallySpacedRectSide\",\"uuid\":\"fdf47ade-06a3-4164-a0ae-b5ab8f0b8a55\"},{\"content\":{\"connectorIds\":[\"In4\",\"Out1\",\"Out2\"],\"side\":\"RIGHT\"},\"type\":\"ConnectorPlacement.EquallySpacedRectSide\",\"uuid\":\"e0a966ff-b656-4cbf-a7ff-a400da725053\"},{\"content\":{\"side\":\"TOP\"},\"type\":\"ConnectorPlacement.EquallySpacedRectSide\",\"uuid\":\"151062ed-8c36-492f-8148-99554d7644ec\"},{\"content\":{\"side\":\"BOTTOM\"},\"type\":\"ConnectorPlacement.EquallySpacedRectSide\",\"uuid\":\"8f8a2450-c04a-404e-aef9-a0f993b87536\"}]},\"type\":\"ConnectorPlacement.EquallySpacedConnector\",\"uuid\":\"01811104-26cd-432b-92b8-9bb1e91d8204\"}],\"packageUris\":[\"http://schema.mathworks.com/mf0/Connector/R2020b\"],\"version\":\"1.0\"}"
  Subsystem4 : Subsystem  ReferencedSubsystem=HVDCSTATION  c=HVDC.C*0.1  vc=HVDC.Vdc  L=HVDC.L/5  VRated=base.kV1  SRated=Base.MVA_base_new  t=grid.sensorTime  Ts=Ts
  Sum : Sum  Inputs=|++
  Sum1 : Sum  Inputs=|+-
  Switch : Switch  Criteria=u2 > Threshold  SaturateOnIntegerOverflow=off  InputSameDT=off
  Terminator{1..3,9} (4 alike) : Terminator
  Unit Delay{,1..3} (4 alike) : UnitDelay  SampleTime=-1  HasFrameUpgradeWarning=on
  Voltage Sensor1 : fl_lib/Electrical/Electrical Sensors/Voltage Sensor
  DC : PMIOPort  Side=Left
  inv1 : PMIOPort  Port=2  Side=Right
  P : Outport
  Q : Outport  Port=2
  wires:
  Unit Delay3/1 -> Subsystem3/2(Vabc)
  Subsystem4/6 -> Terminator3/1
  Unit Delay/1 -> Subsystem3/1(Vabc1)
  Subsystem4/5 -> Unit Delay/1
  Subsystem4/4 -> Terminator2/1
  F/1 -> Subsystem3/4(F)
  Subsystem4/3 -> Terminator1/1
  Subsystem4/2 -> Unit Delay3/1
  VRef/1 -> Unit Delay2/1
  PS-Simulink Converter2/1 -> Terminator9/1  "VdcWF1"
  Sum/1 -> Subsystem3/3(Vref)
  PS-Simulink Converter1/1 -> P/1
  PS-Simulink Converter/1 -> Q/1
  Subsystem4/1 -> Gain/1
  Gain/1 -> Sum1/1  "VdcOff"
  Constant/1 -> Sum1/2
  Constant1/1 -> Switch/3
  Switch/1 -> Gain1/1
  Sum1/1 -> Switch/1, Switch/2
  Gain1/1 -> Unit Delay1/1
  Unit Delay1/1 -> Sum/2
  Unit Delay2/1 -> Sum/1
  Subsystem3/2(VabcRef) -> Simulink-PS Converter1/1
  Subsystem3/1(VabcRef1) -> Simulink-PS Converter2/1
  connections:
  Subsystem4/LConn3 -- Voltage Sensor1/LConn1 -- Simscape Bus/LConn1
  Voltage Sensor1/RConn2 -- Subsystem4/LConn5 -- Simscape Bus/LConn3
  Subsystem4/LConn4 -- Simscape Bus/LConn2
  DC/RConn1 -- Simscape Bus/RConn1
  Power Sensor (Three-Phase)/LConn1 -- inv1/RConn1
  Power Sensor (Three-Phase)/RConn1 -- Subsystem4/RConn1
  PS-Simulink Converter2/LConn1 -- Voltage Sensor1/RConn1
  PS-Simulink Converter/LConn1 -- Power Sensor (Three-Phase)/LConn3
  PS-Simulink Converter1/LConn1 -- Power Sensor (Three-Phase)/LConn2
  ERef1/LConn1 -- Subsystem4/LConn6
  Simulink-PS Converter1/RConn1 -- Subsystem4/LConn1
  Simulink-PS Converter2/RConn1 -- Subsystem4/LConn2
